simulink model "AVIC_model"  (R2015b)
settings: Solver=ode45  StartTime=0.0  StopTime=simtime  RelTol=1e-3
values from neighbouring files (symbols this model uses):
  A = 1    [simulation.m]
  a1 = 1    [simulation.m]
  a2 = 3    [simulation.m]
  a3 = 3    [simulation.m]
  Amp1 = Ampl/1000000    (= 134.217728)    [simulation.m]
  b1 = 1    [simulation.m]
  B2 = 8    [simulation.m]
  C = 32    [simulation.m]
  c1 = 1    [simulation.m]
  c2 = 1    [simulation.m]
  c3 = 1    [simulation.m]
  finrad = 2*pi/(N)*f0*clk    [simulation.m]
  FSC = 2^27    (= 134217728)    [simulation.m]
  SAT = 127    [simulation.m]
  Ts = 1/clk    (= 1.62760416667e-07)    [simulation.m]
libraries: simulink x298
(part 1 of 5)
settings Model: Creator=12x2123  LastModifiedBy=yuki
settings DataIOCC: SaveFormat=Array
settings HardwareCC: ProdBitPerPointer=32  ProdLargestAtomicFloat=None  ProdIntDivRoundTo=Undefined  ProdEndianess=Unspecified  ProdWordSize=32  ProdHWDeviceType=32-bit Generic
settings GRTTargetCC: GeneratePreprocessorConditionals=Disable all
settings ConfigComp: CovModelRefEnable=Off

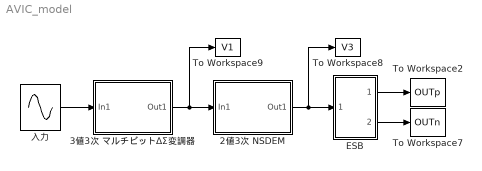
== system AVIC_model ==
  2値3次 NSDEM : Subsystem
  "3値3次 マルチビットΔΣ変調器 " : Subsystem
  ESB : Subsystem
  To Workspace2 : ToWorkspace  VariableName=OUTp  SampleTime=-1
  To Workspace7 : ToWorkspace  VariableName=OUTn  SampleTime=-1
  To Workspace8 : ToWorkspace  VariableName=V3  SampleTime=-1
  To Workspace9 : ToWorkspace  VariableName=V1  SampleTime=-1
  入力 : Sin  Amplitude=Amp1  Frequency=finrad  SampleTime=Ts
  wires:
  入力/1 -> "3値3次 マルチビットΔΣ変調器 "/1(In1)
  "3値3次 マルチビットΔΣ変調器 "/1(Out1) -> To Workspace9/1, 2値3次 NSDEM/1(In1)
  2値3次 NSDEM/1(Out1) -> ESB/1(In1), To Workspace8/1
  ESB/1(Out1) -> To Workspace2/1
  ESB/2(Out2) -> To Workspace7/1

== system AVIC_model/2値3次 NSDEM ==
  In1 : Inport
  NSDEM_3rd : Subsystem
  Out1 : Outport
  wires:
  NSDEM_3rd/1(OUT) -> Out1/1
  In1/1 -> NSDEM_3rd/1(IN)

== system AVIC_model/3値3次 マルチビットΔΣ変調器  ==
  In1 : Inport
  B1 : Gain  Gain=b1  SampleTime=Ts  SaturateOnIntegerOverflow=on  OutDataTypeStr=Inherit: Same as input  ParamDataTypeStr=Inherit: Same as input
  INT1 : Subsystem
  INT2 : Subsystem
  INT3 : Subsystem
  Q1 : Subsystem
  Scope3 : Scope  NumInputPorts=3
  To Workspace1 : ToWorkspace  VariableName=XN  SampleTime=-1
  To Workspace3 : ToWorkspace  VariableName=XN1  SampleTime=-1
  To Workspace4 : ToWorkspace  VariableName=XN2  SampleTime=-1
  To Workspace5 : ToWorkspace  VariableName=V  SampleTime=-1
  To Workspace6 : ToWorkspace  VariableName=Y  SampleTime=-1
  a1 : Gain  Gain=a1  OutDataTypeStr=Inherit: Same as input  ParamDataTypeStr=Inherit: Same as input
  a2 : Gain  Gain=a2  OutDataTypeStr=Inherit: Same as input  ParamDataTypeStr=Inherit: Same as input
  a3 : Gain  Gain=a3  OutDataTypeStr=Inherit: Same as input  ParamDataTypeStr=Inherit: Same as input
  c1 : Gain  Gain=c1  OutDataTypeStr=Inherit: Same as input  ParamDataTypeStr=Inherit: Same as input
  c2 : Gain  Gain=c2  OutDataTypeStr=Inherit: Same as input  ParamDataTypeStr=Inherit: Same as input
  c3 : Gain  Gain=c3  OutDataTypeStr=Inherit: Same as input  ParamDataTypeStr=Inherit: Same as input
  dd : Sum  Inputs=|+-  OutDataTypeStr=double  SaturateOnIntegerOverflow=on  InputSameDT=on
  dd1 : Sum  Inputs=|+-  OutDataTypeStr=double  SaturateOnIntegerOverflow=on  InputSameDT=on
  dd2 : Sum  Inputs=|+-  OutDataTypeStr=double  SaturateOnIntegerOverflow=on  InputSameDT=on
  Out1 : Outport
  wires:
  B1/1 -> dd1/1
  c1/1 -> dd/1
  INT1/1(Out1) -> c1/1, Scope3/1, To Workspace1/1
  a1/1 -> dd1/2
  dd/1 -> INT2/1(In1)
  a2/1 -> dd/2
  Q1/2(DA) -> Out1/1
  dd2/1 -> INT3/1(In1)
  INT2/1(Out1) -> To Workspace3/1, Scope3/2, c2/1
  Q1/1(Out1) -> a3/1, a2/1, a1/1, To Workspace5/1
  c3/1 -> To Workspace6/1, Q1/1(In1)
  dd1/1 -> INT1/1(In1)
  a3/1 -> dd2/2
  c2/1 -> dd2/1
  INT3/1(Out1) -> Scope3/3, To Workspace4/1, c3/1
  In1/1 -> B1/1

== system AVIC_model/ESB ==
  In1 : Inport
  Data Type Conversion2 : DataTypeConversion  OutDataTypeStr=double
  Data Type Conversion3 : DataTypeConversion  OutDataTypeStr=double
  Demux2 : Demux  Outputs=8
  Demux3 : Demux  Outputs=8
  Gain{17..32} (16 alike) : Gain
  Mux : Mux  Inputs=8
  Mux1 : Mux  Inputs=8
  Subsystem4 : Subsystem
  Out1 : Outport
  Out2 : Outport  Port=2
  wires:
  Subsystem4/1(Out1) -> Data Type Conversion2/1
  In1/1 -> Subsystem4/1(In1)
  Demux2/1 -> Gain18/1
  Demux2/2 -> Gain17/1
  Demux2/3 -> Gain20/1
  Demux2/4 -> Gain19/1
  Demux2/5 -> Gain22/1
  Demux2/6 -> Gain21/1
  Demux2/7 -> Gain24/1
  Demux2/8 -> Gain23/1
  Data Type Conversion2/1 -> Demux2/1
  Gain18/1 -> Mux/1
  Gain17/1 -> Mux/2
  Gain20/1 -> Mux/3
  Gain19/1 -> Mux/4
  Gain22/1 -> Mux/5
  Gain23/1 -> Mux/8
  Gain24/1 -> Mux/7
  Gain21/1 -> Mux/6
  Mux/1 -> Out1/1
  Subsystem4/2(Out2) -> Data Type Conversion3/1
  Demux3/1 -> Gain25/1
  Demux3/2 -> Gain32/1
  Demux3/3 -> Gain27/1
  Demux3/4 -> Gain26/1
  Demux3/5 -> Gain29/1
  Demux3/6 -> Gain28/1
  Demux3/7 -> Gain31/1
  Demux3/8 -> Gain30/1
  Data Type Conversion3/1 -> Demux3/1
  Gain25/1 -> Mux1/1
  Gain32/1 -> Mux1/2
  Gain27/1 -> Mux1/3
  Gain26/1 -> Mux1/4
  Gain29/1 -> Mux1/5
  Gain30/1 -> Mux1/8
  Gain31/1 -> Mux1/7
  Gain28/1 -> Mux1/6
  Mux1/1 -> Out2/1

== system AVIC_model/2値3次 NSDEM/NSDEM_3rd ==
  note: SORT8
  IN : Inport
  Data Type Conversion : DataTypeConversion  OutDataTypeStr=double
  Demux : Demux  Outputs=16
  INTEG4_1 : Subsystem
  INTEG4_10 : Subsystem
  INTEG4_11 : Subsystem
  INTEG4_12 : Subsystem
  INTEG4_13 : Subsystem
  INTEG4_14 : Subsystem
  INTEG4_15 : Subsystem
  INTEG4_17 : Subsystem
  INTEG4_2 : Subsystem
  INTEG4_3 : Subsystem
  INTEG4_4 : Subsystem
  INTEG4_5 : Subsystem
  INTEG4_6 : Subsystem
  INTEG4_7 : Subsystem
  INTEG4_8 : Subsystem
  INTEG4_9 : Subsystem
  MinMax : MinMax  Inputs=16
  MinMax1 : MinMax  Inputs=16
  SELECTOR1 : Subsystem
  Scope : Scope  NumInputPorts=16
  Scope1 : Scope  NumInputPorts=16
  Scope2 : Scope  NumInputPorts=16
  Sort16 : Subsystem
  To Workspace1 : ToWorkspace  VariableName=MIN3_1p  SampleTime=-1
  To Workspace2 : ToWorkspace  VariableName=IDX_1p  SampleTime=-1
  To Workspace5 : ToWorkspace  VariableName=MIN1_1p  SampleTime=-1
  To Workspace8 : ToWorkspace  VariableName=MIN2_1p  SampleTime=-1
  OUT : Outport
  wires:
  Sort16/2(IDX) -> To Workspace2/1, SELECTOR1/2(INX)
  Sort16/1(MIN) -> INTEG4_5/4(SUB3), INTEG4_6/4(SUB3), INTEG4_15/4(SUB3), INTEG4_14/4(SUB3), INTEG4_13/4(SUB3), INTEG4_12/4(SUB3), INTEG4_11/4(SUB3), INTEG4_10/4(SUB3), INTEG4_8/4(SUB3), INTEG4_9/4(SUB3), INTEG4_7/4(SUB3), INTEG4_4/4(SUB3), INTEG4_3/4(SUB3), INTEG4_1/4(SUB3), INTEG4_17/4(SUB3), INTEG4_2/4(SUB3), To Workspace1/1
  INTEG4_6/1(OUT1) -> Scope/7, MinMax/7
  INTEG4_5/1(OUT1) -> Scope/6, MinMax/6
  INTEG4_3/1(OUT1) -> Scope/4, MinMax/4
  INTEG4_2/1(OUT1) -> Scope/3, MinMax/3
  INTEG4_1/1(OUT1) -> Scope/2, MinMax/2
  INTEG4_17/1(OUT1) -> Scope/1, MinMax/1
  SELECTOR1/1(SEL) -> Data Type Conversion/1, OUT/1
  IN/1 -> SELECTOR1/1(TH)
  Demux/8 -> INTEG4_7/1(IN)
  Demux/7 -> INTEG4_6/1(IN)
  Demux/6 -> INTEG4_5/1(IN)
  Demux/5 -> INTEG4_4/1(IN)
  Demux/4 -> INTEG4_3/1(IN)
  Demux/3 -> INTEG4_2/1(IN)
  Demux/2 -> INTEG4_1/1(IN)
  Data Type Conversion/1 -> Demux/1
  MinMax1/1 -> INTEG4_17/3(SUB2), INTEG4_1/3(SUB2), INTEG4_2/3(SUB2), INTEG4_3/3(SUB2), INTEG4_4/3(SUB2), INTEG4_5/3(SUB2), INTEG4_6/3(SUB2), INTEG4_15/3(SUB2), INTEG4_14/3(SUB2), INTEG4_13/3(SUB2), INTEG4_12/3(SUB2), INTEG4_11/3(SUB2), INTEG4_10/3(SUB2), INTEG4_8/3(SUB2), INTEG4_9/3(SUB2), INTEG4_7/3(SUB2), To Workspace8/1
  INTEG4_4/1(OUT1) -> Scope/5, MinMax/5
  INTEG4_7/1(OUT1) -> Scope/8, MinMax/8
  Demux/1 -> INTEG4_17/1(IN)
  INTEG4_9/1(OUT1) -> Scope/9, MinMax/9
  INTEG4_8/1(OUT1) -> Scope/10, MinMax/10
  INTEG4_10/1(OUT1) -> Scope/11, MinMax/11
  INTEG4_11/1(OUT1) -> Scope/12, MinMax/12
  INTEG4_12/1(OUT1) -> Scope/13, MinMax/13
  INTEG4_13/1(OUT1) -> Scope/14, MinMax/14
  INTEG4_15/1(OUT1) -> Scope/16, MinMax/16
  Demux/9 -> INTEG4_9/1(IN)
  Demux/10 -> INTEG4_8/1(IN)
  Demux/11 -> INTEG4_10/1(IN)
  Demux/12 -> INTEG4_11/1(IN)
  Demux/16 -> INTEG4_15/1(IN)
  Demux/15 -> INTEG4_14/1(IN)
  Demux/14 -> INTEG4_13/1(IN)
  Demux/13 -> INTEG4_12/1(IN)
  MinMax/1 -> To Workspace5/1, INTEG4_17/2(SUB1), INTEG4_1/2(SUB1), INTEG4_2/2(SUB1), INTEG4_3/2(SUB1), INTEG4_4/2(SUB1), INTEG4_5/2(SUB1), INTEG4_6/2(SUB1), INTEG4_9/2(SUB1), INTEG4_8/2(SUB1), INTEG4_12/2(SUB1), INTEG4_14/2(SUB1), INTEG4_15/2(SUB1), INTEG4_13/2(SUB1), INTEG4_11/2(SUB1), INTEG4_10/2(SUB1), INTEG4_7/2(SUB1)
  INTEG4_14/1(OUT1) -> Scope/15, MinMax/15
  INTEG4_6/2(OUT2) -> Scope1/7, MinMax1/7
  INTEG4_5/2(OUT2) -> Scope1/6, MinMax1/6
  INTEG4_3/2(OUT2) -> Scope1/4, MinMax1/4
  INTEG4_2/2(OUT2) -> Scope1/3, MinMax1/3
  INTEG4_1/2(OUT2) -> Scope1/2, MinMax1/2
  INTEG4_17/2(OUT2) -> Scope1/1, MinMax1/1
  INTEG4_4/2(OUT2) -> Scope1/5, MinMax1/5
  INTEG4_7/2(OUT2) -> Scope1/8, MinMax1/8
  INTEG4_9/2(OUT2) -> Scope1/9, MinMax1/9
  INTEG4_8/2(OUT2) -> Scope1/10, MinMax1/10
  INTEG4_10/2(OUT2) -> Scope1/11, MinMax1/11
  INTEG4_11/2(OUT2) -> Scope1/12, MinMax1/12
  INTEG4_12/2(OUT2) -> Scope1/13, MinMax1/13
  INTEG4_13/2(OUT2) -> Scope1/14, MinMax1/14
  INTEG4_15/2(OUT2) -> Scope1/16, MinMax1/16
  INTEG4_14/2(OUT2) -> Scope1/15, MinMax1/15
  INTEG4_6/3(OUT3) -> Scope2/7, Sort16/7(IN6)
  INTEG4_5/3(OUT3) -> Scope2/6, Sort16/6(IN5)
  INTEG4_3/3(OUT3) -> Scope2/4, Sort16/4(IN3)
  INTEG4_2/3(OUT3) -> Scope2/3, Sort16/3(IN2)
  INTEG4_1/3(OUT3) -> Scope2/2, Sort16/2(IN1)
  INTEG4_17/3(OUT3) -> Scope2/1, Sort16/1(IN0)
  INTEG4_4/3(OUT3) -> Scope2/5, Sort16/5(IN4)
  INTEG4_7/3(OUT3) -> Scope2/8, Sort16/8(IN7)
  INTEG4_9/3(OUT3) -> Scope2/9, Sort16/9(IN8)
  INTEG4_8/3(OUT3) -> Scope2/10, Sort16/10(IN9)
  INTEG4_10/3(OUT3) -> Scope2/11, Sort16/11(IN10)
  INTEG4_11/3(OUT3) -> Scope2/12, Sort16/12(IN11)
  INTEG4_12/3(OUT3) -> Scope2/13, Sort16/13(IN12)
  INTEG4_13/3(OUT3) -> Scope2/14, Sort16/14(IN13)
  INTEG4_15/3(OUT3) -> Scope2/16, Sort16/16(IN15)
  INTEG4_14/3(OUT3) -> Scope2/15, Sort16/15(IN14)

== system AVIC_model/3値3次 マルチビットΔΣ変調器 /INT1 ==
  In1 : Inport
  INT1 : UnitDelay  SampleTime=Ts
  dd2 : Sum  Inputs=++|  OutDataTypeStr=double  SaturateOnIntegerOverflow=on  InputSameDT=on
  Out1 : Outport
  wires:
  dd2/1 -> INT1/1
  INT1/1 -> dd2/1, Out1/1
  In1/1 -> dd2/2

== system AVIC_model/3値3次 マルチビットΔΣ変調器 /INT2 ==
  In1 : Inport
  INT1 : UnitDelay  SampleTime=Ts
  dd2 : Sum  Inputs=++|  OutDataTypeStr=double  SaturateOnIntegerOverflow=on  InputSameDT=on
  Out1 : Outport
  wires:
  In1/1 -> dd2/2
  INT1/1 -> Out1/1, dd2/1
  dd2/1 -> INT1/1

== system AVIC_model/3値3次 マルチビットΔΣ変調器 /INT3 ==
  In1 : Inport
  INT1 : UnitDelay  SampleTime=Ts
  dd2 : Sum  Inputs=++|  OutDataTypeStr=double  SaturateOnIntegerOverflow=on  InputSameDT=on
  Out1 : Outport
  wires:
  dd2/1 -> INT1/1
  INT1/1 -> dd2/1, Out1/1
  In1/1 -> dd2/2

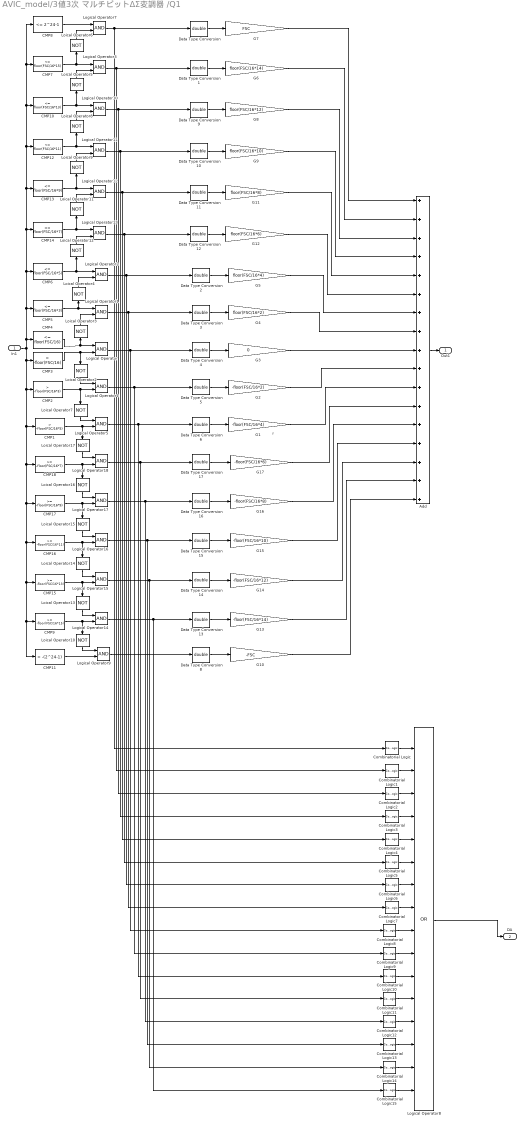
== system AVIC_model/3値3次 マルチビットΔΣ変調器 /Q1 ==
  note: f
  In1 : Inport
  Add : Sum  Inputs=+++++++++++++++++  OutDataTypeStr=double
  CMP1 : simulink/Logic and Bit Operations/Compare To Constant  relop=>  const=-floor(FSC/16*5)  OutDataTypeStr=boolean  ZeroCross=off
  CMP10 : simulink/Logic and Bit Operations/Compare To Constant  relop=<=  const=floor(FSC/16*13)  OutDataTypeStr=boolean  ZeroCross=off
  CMP11 : simulink/Logic and Bit Operations/Compare To Constant  relop=>  const=-(2^24-1)  OutDataTypeStr=boolean  ZeroCross=off
  CMP12 : simulink/Logic and Bit Operations/Compare To Constant  relop=<=  const=floor(FSC/16*11)  OutDataTypeStr=boolean  ZeroCross=off
  CMP13 : simulink/Logic and Bit Operations/Compare To Constant  relop=<=  const=floor(FSC/16*9)  OutDataTypeStr=boolean  ZeroCross=off
  CMP14 : simulink/Logic and Bit Operations/Compare To Constant  relop=<=  const=floor(FSC/16*7)  OutDataTypeStr=boolean  ZeroCross=off
  CMP15 : simulink/Logic and Bit Operations/Compare To Constant  relop=>=  const=-floor(FSC/16*13)  OutDataTypeStr=boolean  ZeroCross=off
  CMP16 : simulink/Logic and Bit Operations/Compare To Constant  relop=>=  const=-floor(FSC/16*11)  OutDataTypeStr=boolean  ZeroCross=off
  CMP17 : simulink/Logic and Bit Operations/Compare To Constant  relop=>=  const=-floor(FSC/16*9)  OutDataTypeStr=boolean  ZeroCross=off
  CMP18 : simulink/Logic and Bit Operations/Compare To Constant  relop=>=  const=-floor(FSC/16*7)  OutDataTypeStr=boolean  ZeroCross=off
  CMP2 : simulink/Logic and Bit Operations/Compare To Constant  relop=>  const=-floor(FSC/16*3)  OutDataTypeStr=boolean  ZeroCross=off
  CMP3 : simulink/Logic and Bit Operations/Compare To Constant  relop=>  const=-floor(FSC/16)  OutDataTypeStr=boolean  ZeroCross=off
  CMP4 : simulink/Logic and Bit Operations/Compare To Constant  relop=<=  const=floor(FSC/16)  OutDataTypeStr=boolean  ZeroCross=off
  CMP5 : simulink/Logic and Bit Operations/Compare To Constant  relop=<=  const=floor(FSC/16*3)  OutDataTypeStr=boolean  ZeroCross=off
  CMP6 : simulink/Logic and Bit Operations/Compare To Constant  relop=<=  const=floor(FSC/16*5)  OutDataTypeStr=boolean  ZeroCross=off
  CMP7 : simulink/Logic and Bit Operations/Compare To Constant  relop=<=  const=floor(FSC/16*15)  OutDataTypeStr=boolean  ZeroCross=off
  CMP8 : simulink/Logic and Bit Operations/Compare To Constant  relop=<=  const=2^24-1  OutDataTypeStr=boolean  ZeroCross=off
  CMP9 : simulink/Logic and Bit Operations/Compare To Constant  relop=>=  const=-floor(FSC/16*15)  OutDataTypeStr=boolean  ZeroCross=off
  Combinatorial Logic : CombinatorialLogic  TruthTable=[0 0 0 0 0 0 0 0 0 0 0 0 0 0 0 0;1 1 1 1 1 1 1 1 1 1 1 1 1 1 1 1]
  Combinatorial Logic1 : CombinatorialLogic  TruthTable=[0 0 0 0 0 0 0 0 0 0 0 0 0 0 0 0;1 1 1 1 1 1 1 1 1 1 1 1 1 1 1 0]
  Combinatorial Logic10 : CombinatorialLogic  TruthTable=[0 0 0 0 0 0 0 0 0 0 0 0 0 0 0 0;1 1 1 1 1 1 0 0 0 0 0 0 0 0 0 0]
  Combinatorial Logic11 : CombinatorialLogic  TruthTable=[0 0 0 0 0 0 0 0 0 0 0 0 0 0 0 0;1 1 1 1 1 0 0 0 0 0 0 0 0 0 0 0]
  Combinatorial Logic12 : CombinatorialLogic  TruthTable=[0 0 0 0 0 0 0 0 0 0 0 0 0 0 0 0;1 1 1 1 0 0 0 0 0 0 0 0 0 0 0 0]
  Combinatorial Logic13 : CombinatorialLogic  TruthTable=[0 0 0 0 0 0 0 0 0 0 0 0 0 0 0 0;1 1 1 0 0 0 0 0 0 0 0 0 0 0 0 0]
  Combinatorial Logic14 : CombinatorialLogic  TruthTable=[0 0 0 0 0 0 0 0 0 0 0 0 0 0 0 0;1 1 0 0 0 0 0 0 0 0 0 0 0 0 0 0]
  Combinatorial Logic15 : CombinatorialLogic  TruthTable=[0 0 0 0 0 0 0 0 0 0 0 0 0 0 0 0;1 0 0 0 0 0 0 0 0 0 0 0 0 0 0 0]
  Combinatorial Logic2 : CombinatorialLogic  TruthTable=[0 0 0 0 0 0 0 0 0 0 0 0 0 0 0 0;1 1 1 1 1 1 1 1 1 1 1 1 1 1 0 0]
  Combinatorial Logic3 : CombinatorialLogic  TruthTable=[0 0 0 0 0 0 0 0 0 0 0 0 0 0 0 0;1 1 1 1 1 1 1 1 1 1 1 1 1 0 0 0]
  Combinatorial Logic4 : CombinatorialLogic  TruthTable=[0 0 0 0 0 0 0 0 0 0 0 0 0 0 0 0;1 1 1 1 1 1 1 1 1 1 1 1 0 0 0 0]
  Combinatorial Logic5 : CombinatorialLogic  TruthTable=[0 0 0 0 0 0 0 0 0 0 0 0 0 0 0 0;1 1 1 1 1 1 1 1 1 1 1 0 0 0 0 0]
  Combinatorial Logic6 : CombinatorialLogic  TruthTable=[0 0 0 0 0 0 0 0 0 0 0 0 0 0 0 0;1 1 1 1 1 1 1 1 1 1 0 0 0 0 0 0]
  Combinatorial Logic7 : CombinatorialLogic  TruthTable=[0 0 0 0 0 0 0 0 0 0 0 0 0 0 0 0;1 1 1 1 1 1 1 1 1 0 0 0 0 0 0 0]
  Combinatorial Logic8 : CombinatorialLogic  TruthTable=[0 0 0 0 0 0 0 0 0 0 0 0 0 0 0 0;1 1 1 1 1 1 1 1 0 0 0 0 0 0 0 0]
  Combinatorial Logic9 : CombinatorialLogic  TruthTable=[0 0 0 0 0 0 0 0 0 0 0 0 0 0 0 0;1 1 1 1 1 1 1 0 0 0 0 0 0 0 0 0]
  Data Type Conversion{,1..6,8..17} (17 alike) : DataTypeConversion  OutDataTypeStr=double
  G1 : Gain  Gain=-floor(FSC/16*4)  OutDataTypeStr=Inherit: Same as input  ParamDataTypeStr=Inherit: Same as input
  G10 : Gain  Gain=-FSC  OutDataTypeStr=Inherit: Same as input  ParamDataTypeStr=Inherit: Same as input
  G11 : Gain  Gain=floor(FSC/16*8)  OutDataTypeStr=Inherit: Same as input  ParamDataTypeStr=Inherit: Same as input
  G12 : Gain  Gain=floor(FSC/16*6)  OutDataTypeStr=Inherit: Same as input  ParamDataTypeStr=Inherit: Same as input
  G13 : Gain  Gain=-floor(FSC/16*14)  OutDataTypeStr=Inherit: Same as input  ParamDataTypeStr=Inherit: Same as input
  G14 : Gain  Gain=-floor(FSC/16*12)  OutDataTypeStr=Inherit: Same as input  ParamDataTypeStr=Inherit: Same as input
  G15 : Gain  Gain=-floor(FSC/16*10)  OutDataTypeStr=Inherit: Same as input  ParamDataTypeStr=Inherit: Same as input
  G16 : Gain  Gain=-floor(FSC/16*8)  OutDataTypeStr=Inherit: Same as input  ParamDataTypeStr=Inherit: Same as input
  G17 : Gain  Gain=-floor(FSC/16*6)  OutDataTypeStr=Inherit: Same as input  ParamDataTypeStr=Inherit: Same as input
  G2 : Gain  Gain=-floor(FSC/16*2)  OutDataTypeStr=Inherit: Same as input  ParamDataTypeStr=Inherit: Same as input
  G3 : Gain  Gain=0  OutDataTypeStr=Inherit: Same as input  ParamDataTypeStr=Inherit: Same as input
  G4 : Gain  Gain=floor(FSC/16*2)  OutDataTypeStr=Inherit: Same as input  ParamDataTypeStr=Inherit: Same as input
  G5 : Gain  Gain=floor(FSC/16*4)  OutDataTypeStr=Inherit: Same as input  ParamDataTypeStr=Inherit: Same as input
  G6 : Gain  Gain=floor(FSC/16*14)  OutDataTypeStr=Inherit: Same as input  ParamDataTypeStr=Inherit: Same as input
  G7 : Gain  Gain=FSC  OutDataTypeStr=Inherit: Same as input  ParamDataTypeStr=Inherit: Same as input
  G8 : Gain  Gain=floor(FSC/16*12)  OutDataTypeStr=Inherit: Same as input  ParamDataTypeStr=Inherit: Same as input
  G9 : Gain  Gain=floor(FSC/16*10)  OutDataTypeStr=Inherit: Same as input  ParamDataTypeStr=Inherit: Same as input
  Logical Operator{,1..5,7,9..18} (17 alike) : Logic  AllPortsSameDT=off  OutDataTypeStr=boolean
  Logical Operator8 : Logic  Operator=OR  Inputs=16  AllPortsSameDT=off  OutDataTypeStr=boolean
  Loical Operator{2..17} (16 alike) : Logic  Operator=NOT  AllPortsSameDT=off  OutDataTypeStr=boolean
  Out1 : Outport
  DA : Outport  Port=2
  wires:
  Combinatorial Logic8/1 -> Logical Operator8/9
  Combinatorial Logic9/1 -> Logical Operator8/10
  Combinatorial Logic10/1 -> Logical Operator8/11
  Combinatorial Logic11/1 -> Logical Operator8/12
  Combinatorial Logic12/1 -> Logical Operator8/13
  Combinatorial Logic13/1 -> Logical Operator8/14
  Combinatorial Logic14/1 -> Logical Operator8/15
  Combinatorial Logic15/1 -> Logical Operator8/16
  Logical Operator8/1 -> DA/1
  Combinatorial Logic/1 -> Logical Operator8/1
  Combinatorial Logic1/1 -> Logical Operator8/2
  Combinatorial Logic2/1 -> Logical Operator8/3
  Combinatorial Logic3/1 -> Logical Operator8/4
  Combinatorial Logic4/1 -> Logical Operator8/5
  Combinatorial Logic5/1 -> Logical Operator8/6
  Combinatorial Logic6/1 -> Logical Operator8/7
  Combinatorial Logic7/1 -> Logical Operator8/8
  G10/1 -> Add/17
  G13/1 -> Add/16
  G14/1 -> Add/15
  G15/1 -> Add/14
  G16/1 -> Add/13
  G17/1 -> Add/12
  G1/1 -> Add/11
  G2/1 -> Add/10
  G3/1 -> Add/9
  G4/1 -> Add/8
  G5/1 -> Add/7
  G12/1 -> Add/6
  G11/1 -> Add/5
  G9/1 -> Add/4
  G8/1 -> Add/3
  G6/1 -> Add/2
  G7/1 -> Add/1
  Data Type Conversion17/1 -> G17/1
  CMP18/1 -> Loical Operator16/1, Logical Operator18/2
  Logical Operator18/1 -> Combinatorial Logic11/1, Data Type Conversion17/1
  Loical Operator17/1 -> Logical Operator18/1
  Data Type Conversion16/1 -> G16/1
  CMP17/1 -> Loical Operator15/1, Logical Operator17/2
  Logical Operator17/1 -> Combinatorial Logic12/1, Data Type Conversion16/1
  Loical Operator16/1 -> Logical Operator17/1
  Data Type Conversion15/1 -> G15/1
  CMP16/1 -> Loical Operator14/1, Logical Operator16/2
  Logical Operator16/1 -> Data Type Conversion15/1, Combinatorial Logic13/1
  Loical Operator15/1 -> Logical Operator16/1
  Data Type Conversion14/1 -> G14/1
  CMP15/1 -> Loical Operator13/1, Logical Operator15/2
  Logical Operator15/1 -> Combinatorial Logic14/1, Data Type Conversion14/1
  Loical Operator14/1 -> Logical Operator15/1
  Data Type Conversion13/1 -> G13/1
  CMP9/1 -> Loical Operator10/1, Logical Operator14/2
  Logical Operator14/1 -> Combinatorial Logic15/1, Data Type Conversion13/1
  Loical Operator13/1 -> Logical Operator14/1
  Data Type Conversion8/1 -> G10/1
  CMP11/1 -> Logical Operator9/2
  Logical Operator9/1 -> Data Type Conversion8/1
  Loical Operator10/1 -> Logical Operator9/1
  Data Type Conversion12/1 -> G12/1
  Logical Operator13/1 -> Combinatorial Logic5/1, Data Type Conversion12/1
  Loical Operator12/1 -> Logical Operator13/2
  CMP14/1 -> Loical Operator11/1, Logical Operator13/1
  Data Type Conversion11/1 -> G11/1
  Logical Operator12/1 -> Combinatorial Logic4/1, Data Type Conversion11/1
  Loical Operator11/1 -> Logical Operator12/2
  CMP13/1 -> Loical Operator9/1, Logical Operator12/1
  Data Type Conversion10/1 -> G9/1
  Logical Operator11/1 -> Combinatorial Logic3/1, Data Type Conversion10/1
  Loical Operator9/1 -> Logical Operator11/2
  CMP12/1 -> Loical Operator8/1, Logical Operator11/1
  Data Type Conversion9/1 -> G8/1
  Logical Operator10/1 -> Combinatorial Logic2/1, Data Type Conversion9/1
  Loical Operator8/1 -> Logical Operator10/2
  CMP10/1 -> Loical Operator5/1, Logical Operator10/1
  Add/1 -> Out1/1
  Data Type Conversion6/1 -> G1/1
  Data Type Conversion5/1 -> G2/1
  Data Type Conversion4/1 -> G3/1
  Data Type Conversion3/1 -> G4/1
  Data Type Conversion2/1 -> G5/1
  Data Type Conversion1/1 -> G6/1
  Data Type Conversion/1 -> G7/1
  Logical Operator7/1 -> Combinatorial Logic/1, Data Type Conversion/1
  Loical Operator6/1 -> Logical Operator7/2
  CMP8/1 -> Logical Operator7/1
  In1/1 -> CMP9/1, CMP11/1, CMP15/1, CMP16/1, CMP17/1, CMP18/1, CMP1/1, CMP2/1, CMP3/1, CMP4/1, CMP7/1, CMP8/1, CMP10/1, CMP12/1, CMP13/1, CMP14/1, CMP6/1, CMP5/1
  CMP3/1 -> Logical Operator/2, Loical Operator2/1
  CMP2/1 -> Logical Operator4/2, Loical Operator7/1
  CMP1/1 -> Loical Operator17/1, Logical Operator5/2
  Logical Operator3/1 -> Combinatorial Logic1/1, Data Type Conversion1/1
  Logical Operator2/1 -> Combinatorial Logic6/1, Data Type Conversion2/1
  Logical Operator1/1 -> Combinatorial Logic7/1, Data Type Conversion3/1
  Logical Operator/1 -> Combinatorial Logic8/1, Data Type Conversion4/1
  Logical Operator4/1 -> Combinatorial Logic9/1, Data Type Conversion5/1
  Logical Operator5/1 -> Combinatorial Logic10/1, Data Type Conversion6/1
  Loical Operator7/1 -> Logical Operator5/1
  Loical Operator2/1 -> Logical Operator4/1
  CMP4/1 -> Logical Operator/1, Loical Operator3/1
  Loical Operator3/1 -> Logical Operator1/2
  CMP5/1 -> Logical Operator1/1, Loical Operator4/1
  Loical Operator4/1 -> Logical Operator2/2
  CMP6/1 -> Loical Operator12/1, Logical Operator2/1
  Loical Operator5/1 -> Logical Operator3/2
  CMP7/1 -> Loical Operator6/1, Logical Operator3/1

== system AVIC_model/ESB/Subsystem4 ==
  In1 : Inport
  Demux : Demux  Outputs=16
  Logical Operator : Logic  Operator=OR  Inputs=8  AllPortsSameDT=off  OutDataTypeStr=boolean
  Logical Operator1 : Logic  Operator=OR  Inputs=8  AllPortsSameDT=off  OutDataTypeStr=boolean
  Subsystem : Subsystem
  Subsystem1 : Subsystem
  Subsystem2 : Subsystem
  Subsystem3 : Subsystem
  Subsystem4 : Subsystem
  Subsystem5 : Subsystem
  Subsystem6 : Subsystem
  Subsystem7 : Subsystem
  Sum{,1..7} (8 alike) : Sum
  To Workspace2 : ToWorkspace  VariableName=OUTp1  SampleTime=-1
  To Workspace7 : ToWorkspace  VariableName=OUTn1  SampleTime=-1
  Out1 : Outport
  Out2 : Outport  Port=2
  wires:
  In1/1 -> Demux/1
  Logical Operator/1 -> Out1/1
  Logical Operator1/1 -> Out2/1
  Sum1/1 -> Subsystem1/1(In1)
  Sum2/1 -> Subsystem2/1(In1)
  Sum/1 -> Subsystem/1(In1)
  Sum3/1 -> Subsystem3/1(In1)
  Sum5/1 -> Subsystem5/1(In1)
  Sum6/1 -> Subsystem6/1(In1)
  Sum4/1 -> Subsystem4/1(In1)
  Sum7/1 -> Subsystem7/1(In1)
  Demux/1 -> Sum/1
  Demux/2 -> Sum/2
  Demux/3 -> Sum1/1
  Demux/4 -> Sum1/2
  Demux/5 -> Sum2/1
  Demux/6 -> Sum2/2
  Demux/7 -> Sum3/1
  Demux/8 -> Sum3/2
  Demux/9 -> Sum4/1
  Demux/10 -> Sum4/2
  Demux/11 -> Sum5/1
  Demux/12 -> Sum5/2
  Demux/13 -> Sum6/1
  Demux/14 -> Sum6/2
  Demux/15 -> Sum7/1
  Demux/16 -> Sum7/2
  Subsystem/1("P1 ") -> Logical Operator/1, To Workspace2/1
  Subsystem1/1("P1 ") -> Logical Operator/2
  Subsystem2/1("P1 ") -> Logical Operator/3
  Subsystem3/1("P1 ") -> Logical Operator/4
  Subsystem4/1("P1 ") -> Logical Operator/5
  Subsystem5/1("P1 ") -> Logical Operator/6
  Subsystem6/1("P1 ") -> Logical Operator/7
  Subsystem7/1("P1 ") -> Logical Operator/8
  Subsystem/2("N1 ") -> To Workspace7/1, Logical Operator1/1
  Subsystem1/2("N1 ") -> Logical Operator1/2
  Subsystem2/2("N1 ") -> Logical Operator1/3
  Subsystem3/2("N1 ") -> Logical Operator1/4
  Subsystem4/2("N1 ") -> Logical Operator1/5
  Subsystem5/2("N1 ") -> Logical Operator1/6
  Subsystem6/2("N1 ") -> Logical Operator1/7
  Subsystem7/2("N1 ") -> Logical Operator1/8

== system AVIC_model/2値3次 NSDEM/NSDEM_3rd/INTEG4_1 ==
  IN : Inport
  SUB1 : Inport  Port=2
  SUB2 : Inport  Port=3
  SUB3 : Inport  Port=4
  Add{1..5} (5 alike) : Sum  Inputs=++-
  Gain : Gain  Gain=B2
  Gain1 : Gain  Gain=A
  Gain2 : Gain  Gain=C
  INT1 : UnitDelay  SampleTime=Ts
  INT2 : UnitDelay  SampleTime=Ts
  INT3 : UnitDelay  SampleTime=Ts
  Saturation{,1..4} (5 alike) : Saturate  UpperLimit=SAT  LowerLimit=-SAT
  OUT1 : Outport
  OUT2 : Outport  Port=2
  OUT3 : Outport  Port=3
  wires:
  SUB3/1 -> Add2/3
  INT1/1 -> Add2/1, OUT3/1
  INT2/1 -> OUT1/1, Add4/1, Add1/2
  Add4/1 -> Saturation/1
  SUB1/1 -> Add4/3, Add1/3
  IN/1 -> Gain/1, Gain2/1, Gain1/1
  Add1/1 -> Saturation1/1
  Gain/1 -> Add1/1
  Add2/1 -> Saturation2/1
  Saturation/1 -> INT2/1
  Saturation2/1 -> INT1/1
  INT3/1 -> OUT2/1, Add5/1, Add3/2
  Add5/1 -> Saturation3/1
  SUB2/1 -> Add5/3, Add3/3
  Add3/1 -> Saturation4/1
  Gain2/1 -> Add3/1
  Saturation3/1 -> INT3/1
  Saturation4/1 -> Add2/2
  Saturation1/1 -> Add5/2
  Gain1/1 -> Add4/2

== system AVIC_model/2値3次 NSDEM/NSDEM_3rd/INTEG4_10 ==
  IN : Inport
  SUB1 : Inport  Port=2
  SUB2 : Inport  Port=3
  SUB3 : Inport  Port=4
  Add{1..5} (5 alike) : Sum  Inputs=++-
  Gain : Gain  Gain=B2
  Gain1 : Gain  Gain=A
  Gain2 : Gain  Gain=C
  INT1 : UnitDelay  SampleTime=Ts
  INT2 : UnitDelay  SampleTime=Ts
  INT3 : UnitDelay  SampleTime=Ts
  Saturation{,1..4} (5 alike) : Saturate  UpperLimit=SAT  LowerLimit=-SAT
  OUT1 : Outport
  OUT2 : Outport  Port=2
  OUT3 : Outport  Port=3
  wires:
  SUB3/1 -> Add2/3
  INT1/1 -> Add2/1, OUT3/1
  INT2/1 -> OUT1/1, Add4/1, Add1/2
  Add4/1 -> Saturation/1
  SUB1/1 -> Add4/3, Add1/3
  IN/1 -> Gain/1, Gain2/1, Gain1/1
  Add1/1 -> Saturation1/1
  Gain/1 -> Add1/1
  Add2/1 -> Saturation2/1
  Saturation/1 -> INT2/1
  Saturation2/1 -> INT1/1
  INT3/1 -> OUT2/1, Add5/1, Add3/2
  Add5/1 -> Saturation3/1
  SUB2/1 -> Add5/3, Add3/3
  Add3/1 -> Saturation4/1
  Gain2/1 -> Add3/1
  Saturation3/1 -> INT3/1
  Saturation4/1 -> Add2/2
  Saturation1/1 -> Add5/2
  Gain1/1 -> Add4/2

== system AVIC_model/2値3次 NSDEM/NSDEM_3rd/INTEG4_11 ==
  IN : Inport
  SUB1 : Inport  Port=2
  SUB2 : Inport  Port=3
  SUB3 : Inport  Port=4
  Add{1..5} (5 alike) : Sum  Inputs=++-
  Gain : Gain  Gain=B2
  Gain1 : Gain  Gain=A
  Gain2 : Gain  Gain=C
  INT1 : UnitDelay  SampleTime=Ts
  INT2 : UnitDelay  SampleTime=Ts
  INT3 : UnitDelay  SampleTime=Ts
  Saturation{,1..4} (5 alike) : Saturate  UpperLimit=SAT  LowerLimit=-SAT
  OUT1 : Outport
  OUT2 : Outport  Port=2
  OUT3 : Outport  Port=3
  wires:
  SUB3/1 -> Add2/3
  INT1/1 -> Add2/1, OUT3/1
  INT2/1 -> OUT1/1, Add4/1, Add1/2
  Add4/1 -> Saturation/1
  SUB1/1 -> Add4/3, Add1/3
  IN/1 -> Gain/1, Gain2/1, Gain1/1
  Add1/1 -> Saturation1/1
  Gain/1 -> Add1/1
  Add2/1 -> Saturation2/1
  Saturation/1 -> INT2/1
  Saturation2/1 -> INT1/1
  INT3/1 -> OUT2/1, Add5/1, Add3/2
  Add5/1 -> Saturation3/1
  SUB2/1 -> Add5/3, Add3/3
  Add3/1 -> Saturation4/1
  Gain2/1 -> Add3/1
  Saturation3/1 -> INT3/1
  Saturation4/1 -> Add2/2
  Saturation1/1 -> Add5/2
  Gain1/1 -> Add4/2

== system AVIC_model/2値3次 NSDEM/NSDEM_3rd/INTEG4_12 ==
  IN : Inport
  SUB1 : Inport  Port=2
  SUB2 : Inport  Port=3
  SUB3 : Inport  Port=4
  Add{1..5} (5 alike) : Sum  Inputs=++-
  Gain : Gain  Gain=B2
  Gain1 : Gain  Gain=A
  Gain2 : Gain  Gain=C
  INT1 : UnitDelay  SampleTime=Ts
  INT2 : UnitDelay  SampleTime=Ts
  INT3 : UnitDelay  SampleTime=Ts
  Saturation{,1..4} (5 alike) : Saturate  UpperLimit=SAT  LowerLimit=-SAT
  OUT1 : Outport
  OUT2 : Outport  Port=2
  OUT3 : Outport  Port=3
  wires:
  SUB3/1 -> Add2/3
  INT1/1 -> Add2/1, OUT3/1
  INT2/1 -> OUT1/1, Add4/1, Add1/2
  Add4/1 -> Saturation/1
  SUB1/1 -> Add4/3, Add1/3
  IN/1 -> Gain/1, Gain2/1, Gain1/1
  Add1/1 -> Saturation1/1
  Gain/1 -> Add1/1
  Add2/1 -> Saturation2/1
  Saturation/1 -> INT2/1
  Saturation2/1 -> INT1/1
  INT3/1 -> OUT2/1, Add5/1, Add3/2
  Add5/1 -> Saturation3/1
  SUB2/1 -> Add5/3, Add3/3
  Add3/1 -> Saturation4/1
  Gain2/1 -> Add3/1
  Saturation3/1 -> INT3/1
  Saturation4/1 -> Add2/2
  Saturation1/1 -> Add5/2
  Gain1/1 -> Add4/2

== system AVIC_model/2値3次 NSDEM/NSDEM_3rd/INTEG4_13 ==
  IN : Inport
  SUB1 : Inport  Port=2
  SUB2 : Inport  Port=3
  SUB3 : Inport  Port=4
  Add{1..5} (5 alike) : Sum  Inputs=++-
  Gain : Gain  Gain=B2
  Gain1 : Gain  Gain=A
  Gain2 : Gain  Gain=C
  INT1 : UnitDelay  SampleTime=Ts
  INT2 : UnitDelay  SampleTime=Ts
  INT3 : UnitDelay  SampleTime=Ts
  Saturation{,1..4} (5 alike) : Saturate  UpperLimit=SAT  LowerLimit=-SAT
  OUT1 : Outport
  OUT2 : Outport  Port=2
  OUT3 : Outport  Port=3
  wires:
  SUB3/1 -> Add2/3
  INT1/1 -> Add2/1, OUT3/1
  INT2/1 -> OUT1/1, Add4/1, Add1/2
  Add4/1 -> Saturation/1
  SUB1/1 -> Add4/3, Add1/3
  IN/1 -> Gain/1, Gain2/1, Gain1/1
  Add1/1 -> Saturation1/1
  Gain/1 -> Add1/1
  Add2/1 -> Saturation2/1
  Saturation/1 -> INT2/1
  Saturation2/1 -> INT1/1
  INT3/1 -> OUT2/1, Add5/1, Add3/2
  Add5/1 -> Saturation3/1
  SUB2/1 -> Add5/3, Add3/3
  Add3/1 -> Saturation4/1
  Gain2/1 -> Add3/1
  Saturation3/1 -> INT3/1
  Saturation4/1 -> Add2/2
  Saturation1/1 -> Add5/2
  Gain1/1 -> Add4/2

== system AVIC_model/2値3次 NSDEM/NSDEM_3rd/INTEG4_14 ==
  IN : Inport
  SUB1 : Inport  Port=2
  SUB2 : Inport  Port=3
  SUB3 : Inport  Port=4
  Add{1..5} (5 alike) : Sum  Inputs=++-
  Gain : Gain  Gain=B2
  Gain1 : Gain  Gain=A
  Gain2 : Gain  Gain=C
  INT1 : UnitDelay  SampleTime=Ts
  INT2 : UnitDelay  SampleTime=Ts
  INT3 : UnitDelay  SampleTime=Ts
  Saturation{,1..4} (5 alike) : Saturate  UpperLimit=SAT  LowerLimit=-SAT
  OUT1 : Outport
  OUT2 : Outport  Port=2
  OUT3 : Outport  Port=3
  wires:
  SUB3/1 -> Add2/3
  INT1/1 -> Add2/1, OUT3/1
  INT2/1 -> OUT1/1, Add4/1, Add1/2
  Add4/1 -> Saturation/1
  SUB1/1 -> Add4/3, Add1/3
  IN/1 -> Gain/1, Gain2/1, Gain1/1
  Add1/1 -> Saturation1/1
  Gain/1 -> Add1/1
  Add2/1 -> Saturation2/1
  Saturation/1 -> INT2/1
  Saturation2/1 -> INT1/1
  INT3/1 -> OUT2/1, Add5/1, Add3/2
  Add5/1 -> Saturation3/1
  SUB2/1 -> Add5/3, Add3/3
  Add3/1 -> Saturation4/1
  Gain2/1 -> Add3/1
  Saturation3/1 -> INT3/1
  Saturation4/1 -> Add2/2
  Saturation1/1 -> Add5/2
  Gain1/1 -> Add4/2

== system AVIC_model/2値3次 NSDEM/NSDEM_3rd/INTEG4_15 ==
  IN : Inport
  SUB1 : Inport  Port=2
  SUB2 : Inport  Port=3
  SUB3 : Inport  Port=4
  Add{1..5} (5 alike) : Sum  Inputs=++-
  Gain : Gain  Gain=B2
  Gain1 : Gain  Gain=A
  Gain2 : Gain  Gain=C
  INT1 : UnitDelay  SampleTime=Ts
  INT2 : UnitDelay  SampleTime=Ts
  INT3 : UnitDelay  SampleTime=Ts
  Saturation{,1..4} (5 alike) : Saturate  UpperLimit=SAT  LowerLimit=-SAT
  OUT1 : Outport
  OUT2 : Outport  Port=2
  OUT3 : Outport  Port=3
  wires:
  SUB3/1 -> Add2/3
  INT1/1 -> Add2/1, OUT3/1
  INT2/1 -> OUT1/1, Add4/1, Add1/2
  Add4/1 -> Saturation/1
  SUB1/1 -> Add4/3, Add1/3
  IN/1 -> Gain/1, Gain2/1, Gain1/1
  Add1/1 -> Saturation1/1
  Gain/1 -> Add1/1
  Add2/1 -> Saturation2/1
  Saturation/1 -> INT2/1
  Saturation2/1 -> INT1/1
  INT3/1 -> OUT2/1, Add5/1, Add3/2
  Add5/1 -> Saturation3/1
  SUB2/1 -> Add5/3, Add3/3
  Add3/1 -> Saturation4/1
  Gain2/1 -> Add3/1
  Saturation3/1 -> INT3/1
  Saturation4/1 -> Add2/2
  Saturation1/1 -> Add5/2
  Gain1/1 -> Add4/2

== system AVIC_model/2値3次 NSDEM/NSDEM_3rd/INTEG4_17 ==
  IN : Inport
  SUB1 : Inport  Port=2
  SUB2 : Inport  Port=3
  SUB3 : Inport  Port=4
  Add{1..5} (5 alike) : Sum  Inputs=++-
  Gain : Gain  Gain=B2
  Gain1 : Gain  Gain=A
  Gain2 : Gain  Gain=C
  INT1 : UnitDelay  SampleTime=Ts
  INT2 : UnitDelay  SampleTime=Ts
  INT3 : UnitDelay  SampleTime=Ts
  Saturation{,1..4} (5 alike) : Saturate  UpperLimit=SAT  LowerLimit=-SAT
  OUT1 : Outport
  OUT2 : Outport  Port=2
  OUT3 : Outport  Port=3
  wires:
  SUB3/1 -> Add2/3
  INT1/1 -> Add2/1, OUT3/1
  INT2/1 -> OUT1/1, Add4/1, Add1/2
  Add4/1 -> Saturation/1
  SUB1/1 -> Add4/3, Add1/3
  IN/1 -> Gain/1, Gain2/1, Gain1/1
  Add1/1 -> Saturation1/1
  Gain/1 -> Add1/1
  Add2/1 -> Saturation2/1
  Saturation/1 -> INT2/1
  Saturation2/1 -> INT1/1
  INT3/1 -> OUT2/1, Add5/1, Add3/2
  Add5/1 -> Saturation3/1
  SUB2/1 -> Add5/3, Add3/3
  Add3/1 -> Saturation4/1
  Gain2/1 -> Add3/1
  Saturation3/1 -> INT3/1
  Saturation4/1 -> Add2/2
  Saturation1/1 -> Add5/2
  Gain1/1 -> Add4/2

== system AVIC_model/2値3次 NSDEM/NSDEM_3rd/INTEG4_2 ==
  IN : Inport
  SUB1 : Inport  Port=2
  SUB2 : Inport  Port=3
  SUB3 : Inport  Port=4
  Add{1..5} (5 alike) : Sum  Inputs=++-
  Gain : Gain  Gain=B2
  Gain1 : Gain  Gain=A
  Gain2 : Gain  Gain=C
  INT1 : UnitDelay  SampleTime=Ts
  INT2 : UnitDelay  SampleTime=Ts
  INT3 : UnitDelay  SampleTime=Ts
  Saturation{,1..4} (5 alike) : Saturate  UpperLimit=SAT  LowerLimit=-SAT
  OUT1 : Outport
  OUT2 : Outport  Port=2
  OUT3 : Outport  Port=3
  wires:
  SUB3/1 -> Add2/3
  INT1/1 -> Add2/1, OUT3/1
  INT2/1 -> OUT1/1, Add4/1, Add1/2
  Add4/1 -> Saturation/1
  SUB1/1 -> Add4/3, Add1/3
  IN/1 -> Gain/1, Gain2/1, Gain1/1
  Add1/1 -> Saturation1/1
  Gain/1 -> Add1/1
  Add2/1 -> Saturation2/1
  Saturation/1 -> INT2/1
  Saturation2/1 -> INT1/1
  INT3/1 -> OUT2/1, Add5/1, Add3/2
  Add5/1 -> Saturation3/1
  SUB2/1 -> Add5/3, Add3/3
  Add3/1 -> Saturation4/1
  Gain2/1 -> Add3/1
  Saturation3/1 -> INT3/1
  Saturation4/1 -> Add2/2
  Saturation1/1 -> Add5/2
  Gain1/1 -> Add4/2

== system AVIC_model/2値3次 NSDEM/NSDEM_3rd/INTEG4_3 ==
  IN : Inport
  SUB1 : Inport  Port=2
  SUB2 : Inport  Port=3
  SUB3 : Inport  Port=4
  Add{1..5} (5 alike) : Sum  Inputs=++-
  Gain : Gain  Gain=B2
  Gain1 : Gain  Gain=A
  Gain2 : Gain  Gain=C
  INT1 : UnitDelay  SampleTime=Ts
  INT2 : UnitDelay  SampleTime=Ts
  INT3 : UnitDelay  SampleTime=Ts
  Saturation{,1..4} (5 alike) : Saturate  UpperLimit=SAT  LowerLimit=-SAT
  OUT1 : Outport
  OUT2 : Outport  Port=2
  OUT3 : Outport  Port=3
  wires:
  SUB3/1 -> Add2/3
  INT1/1 -> Add2/1, OUT3/1
  INT2/1 -> OUT1/1, Add4/1, Add1/2
  Add4/1 -> Saturation/1
  SUB1/1 -> Add4/3, Add1/3
  IN/1 -> Gain/1, Gain2/1, Gain1/1
  Add1/1 -> Saturation1/1
  Gain/1 -> Add1/1
  Add2/1 -> Saturation2/1
  Saturation/1 -> INT2/1
  Saturation2/1 -> INT1/1
  INT3/1 -> OUT2/1, Add5/1, Add3/2
  Add5/1 -> Saturation3/1
  SUB2/1 -> Add5/3, Add3/3
  Add3/1 -> Saturation4/1
  Gain2/1 -> Add3/1
  Saturation3/1 -> INT3/1
  Saturation4/1 -> Add2/2
  Saturation1/1 -> Add5/2
  Gain1/1 -> Add4/2

== system AVIC_model/2値3次 NSDEM/NSDEM_3rd/INTEG4_4 ==
  IN : Inport
  SUB1 : Inport  Port=2
  SUB2 : Inport  Port=3
  SUB3 : Inport  Port=4
  Add{1..5} (5 alike) : Sum  Inputs=++-
  Gain : Gain  Gain=B2
  Gain1 : Gain  Gain=A
  Gain2 : Gain  Gain=C
  INT1 : UnitDelay  SampleTime=Ts
  INT2 : UnitDelay  SampleTime=Ts
  INT3 : UnitDelay  SampleTime=Ts
  Saturation{,1..4} (5 alike) : Saturate  UpperLimit=SAT  LowerLimit=-SAT
  OUT1 : Outport
  OUT2 : Outport  Port=2
  OUT3 : Outport  Port=3
  wires:
  SUB3/1 -> Add2/3
  INT1/1 -> Add2/1, OUT3/1
  INT2/1 -> OUT1/1, Add4/1, Add1/2
  Add4/1 -> Saturation/1
  SUB1/1 -> Add4/3, Add1/3
  IN/1 -> Gain/1, Gain2/1, Gain1/1
  Add1/1 -> Saturation1/1
  Gain/1 -> Add1/1
  Add2/1 -> Saturation2/1
  Saturation/1 -> INT2/1
  Saturation2/1 -> INT1/1
  INT3/1 -> OUT2/1, Add5/1, Add3/2
  Add5/1 -> Saturation3/1
  SUB2/1 -> Add5/3, Add3/3
  Add3/1 -> Saturation4/1
  Gain2/1 -> Add3/1
  Saturation3/1 -> INT3/1
  Saturation4/1 -> Add2/2
  Saturation1/1 -> Add5/2
  Gain1/1 -> Add4/2

== system AVIC_model/2値3次 NSDEM/NSDEM_3rd/INTEG4_5 ==
  IN : Inport
  SUB1 : Inport  Port=2
  SUB2 : Inport  Port=3
  SUB3 : Inport  Port=4
  Add{1..5} (5 alike) : Sum  Inputs=++-
  Gain : Gain  Gain=B2
  Gain1 : Gain  Gain=A
  Gain2 : Gain  Gain=C
  INT1 : UnitDelay  SampleTime=Ts
  INT2 : UnitDelay  SampleTime=Ts
  INT3 : UnitDelay  SampleTime=Ts
  Saturation{,1..4} (5 alike) : Saturate  UpperLimit=SAT  LowerLimit=-SAT
  OUT1 : Outport
  OUT2 : Outport  Port=2
  OUT3 : Outport  Port=3
  wires:
  SUB3/1 -> Add2/3
  INT1/1 -> Add2/1, OUT3/1
  INT2/1 -> OUT1/1, Add4/1, Add1/2
  Add4/1 -> Saturation/1
  SUB1/1 -> Add4/3, Add1/3
  IN/1 -> Gain/1, Gain2/1, Gain1/1
  Add1/1 -> Saturation1/1
  Gain/1 -> Add1/1
  Add2/1 -> Saturation2/1
  Saturation/1 -> INT2/1
  Saturation2/1 -> INT1/1
  INT3/1 -> OUT2/1, Add5/1, Add3/2
  Add5/1 -> Saturation3/1
  SUB2/1 -> Add5/3, Add3/3
  Add3/1 -> Saturation4/1
  Gain2/1 -> Add3/1
  Saturation3/1 -> INT3/1
  Saturation4/1 -> Add2/2
  Saturation1/1 -> Add5/2
  Gain1/1 -> Add4/2

== system AVIC_model/2値3次 NSDEM/NSDEM_3rd/INTEG4_6 ==
  IN : Inport
  SUB1 : Inport  Port=2
  SUB2 : Inport  Port=3
  SUB3 : Inport  Port=4
  Add{1..5} (5 alike) : Sum  Inputs=++-
  Gain : Gain  Gain=B2
  Gain1 : Gain  Gain=A
  Gain2 : Gain  Gain=C
  INT1 : UnitDelay  SampleTime=Ts
  INT2 : UnitDelay  SampleTime=Ts
  INT3 : UnitDelay  SampleTime=Ts
  Saturation{,1..4} (5 alike) : Saturate  UpperLimit=SAT  LowerLimit=-SAT
  OUT1 : Outport
  OUT2 : Outport  Port=2
  OUT3 : Outport  Port=3
  wires:
  SUB3/1 -> Add2/3
  INT1/1 -> Add2/1, OUT3/1
  INT2/1 -> OUT1/1, Add4/1, Add1/2
  Add4/1 -> Saturation/1
  SUB1/1 -> Add4/3, Add1/3
  IN/1 -> Gain/1, Gain2/1, Gain1/1
  Add1/1 -> Saturation1/1
  Gain/1 -> Add1/1
  Add2/1 -> Saturation2/1
  Saturation/1 -> INT2/1
  Saturation2/1 -> INT1/1
  INT3/1 -> OUT2/1, Add5/1, Add3/2
  Add5/1 -> Saturation3/1
  SUB2/1 -> Add5/3, Add3/3
  Add3/1 -> Saturation4/1
  Gain2/1 -> Add3/1
  Saturation3/1 -> INT3/1
  Saturation4/1 -> Add2/2
  Saturation1/1 -> Add5/2
  Gain1/1 -> Add4/2

== system AVIC_model/2値3次 NSDEM/NSDEM_3rd/INTEG4_7 ==
  IN : Inport
  SUB1 : Inport  Port=2
  SUB2 : Inport  Port=3
  SUB3 : Inport  Port=4
  Add{1..5} (5 alike) : Sum  Inputs=++-
  Gain : Gain  Gain=B2
  Gain1 : Gain  Gain=A
  Gain2 : Gain  Gain=C
  INT1 : UnitDelay  SampleTime=Ts
  INT2 : UnitDelay  SampleTime=Ts
  INT3 : UnitDelay  SampleTime=Ts
  Saturation{,1..4} (5 alike) : Saturate  UpperLimit=SAT  LowerLimit=-SAT
  OUT1 : Outport
  OUT2 : Outport  Port=2
  OUT3 : Outport  Port=3
  wires:
  SUB3/1 -> Add2/3
  INT1/1 -> Add2/1, OUT3/1
  INT2/1 -> OUT1/1, Add4/1, Add1/2
  Add4/1 -> Saturation/1
  SUB1/1 -> Add4/3, Add1/3
  IN/1 -> Gain/1, Gain2/1, Gain1/1
  Add1/1 -> Saturation1/1
  Gain/1 -> Add1/1
  Add2/1 -> Saturation2/1
  Saturation/1 -> INT2/1
  Saturation2/1 -> INT1/1
  INT3/1 -> OUT2/1, Add5/1, Add3/2
  Add5/1 -> Saturation3/1
  SUB2/1 -> Add5/3, Add3/3
  Add3/1 -> Saturation4/1
  Gain2/1 -> Add3/1
  Saturation3/1 -> INT3/1
  Saturation4/1 -> Add2/2
  Saturation1/1 -> Add5/2
  Gain1/1 -> Add4/2

== system AVIC_model/2値3次 NSDEM/NSDEM_3rd/INTEG4_8 ==
  IN : Inport
  SUB1 : Inport  Port=2
  SUB2 : Inport  Port=3
  SUB3 : Inport  Port=4
  Add{1..5} (5 alike) : Sum  Inputs=++-
  Gain : Gain  Gain=B2
  Gain1 : Gain  Gain=A
  Gain2 : Gain  Gain=C
  INT1 : UnitDelay  SampleTime=Ts
  INT2 : UnitDelay  SampleTime=Ts
  INT3 : UnitDelay  SampleTime=Ts
  Saturation{,1..4} (5 alike) : Saturate  UpperLimit=SAT  LowerLimit=-SAT
  OUT1 : Outport
  OUT2 : Outport  Port=2
  OUT3 : Outport  Port=3
  wires:
  SUB3/1 -> Add2/3
  INT1/1 -> Add2/1, OUT3/1
  INT2/1 -> OUT1/1, Add4/1, Add1/2
  Add4/1 -> Saturation/1
  SUB1/1 -> Add4/3, Add1/3
  IN/1 -> Gain/1, Gain2/1, Gain1/1
  Add1/1 -> Saturation1/1
  Gain/1 -> Add1/1
  Add2/1 -> Saturation2/1
  Saturation/1 -> INT2/1
  Saturation2/1 -> INT1/1
  INT3/1 -> OUT2/1, Add5/1, Add3/2
  Add5/1 -> Saturation3/1
  SUB2/1 -> Add5/3, Add3/3
  Add3/1 -> Saturation4/1
  Gain2/1 -> Add3/1
  Saturation3/1 -> INT3/1
  Saturation4/1 -> Add2/2
  Saturation1/1 -> Add5/2
  Gain1/1 -> Add4/2

== system AVIC_model/2値3次 NSDEM/NSDEM_3rd/INTEG4_9 ==
  IN : Inport
  SUB1 : Inport  Port=2
  SUB2 : Inport  Port=3
  SUB3 : Inport  Port=4
  Add{1..5} (5 alike) : Sum  Inputs=++-
  Gain : Gain  Gain=B2
  Gain1 : Gain  Gain=A
  Gain2 : Gain  Gain=C
  INT1 : UnitDelay  SampleTime=Ts
  INT2 : UnitDelay  SampleTime=Ts
  INT3 : UnitDelay  SampleTime=Ts
  Saturation{,1..4} (5 alike) : Saturate  UpperLimit=SAT  LowerLimit=-SAT
  OUT1 : Outport
  OUT2 : Outport  Port=2
  OUT3 : Outport  Port=3
  wires:
  SUB3/1 -> Add2/3
  INT1/1 -> Add2/1, OUT3/1
  INT2/1 -> OUT1/1, Add4/1, Add1/2
  Add4/1 -> Saturation/1
  SUB1/1 -> Add4/3, Add1/3
  IN/1 -> Gain/1, Gain2/1, Gain1/1
  Add1/1 -> Saturation1/1
  Gain/1 -> Add1/1
  Add2/1 -> Saturation2/1
  Saturation/1 -> INT2/1
  Saturation2/1 -> INT1/1
  INT3/1 -> OUT2/1, Add5/1, Add3/2
  Add5/1 -> Saturation3/1
  SUB2/1 -> Add5/3, Add3/3
  Add3/1 -> Saturation4/1
  Gain2/1 -> Add3/1
  Saturation3/1 -> INT3/1
  Saturation4/1 -> Add2/2
  Saturation1/1 -> Add5/2
  Gain1/1 -> Add4/2

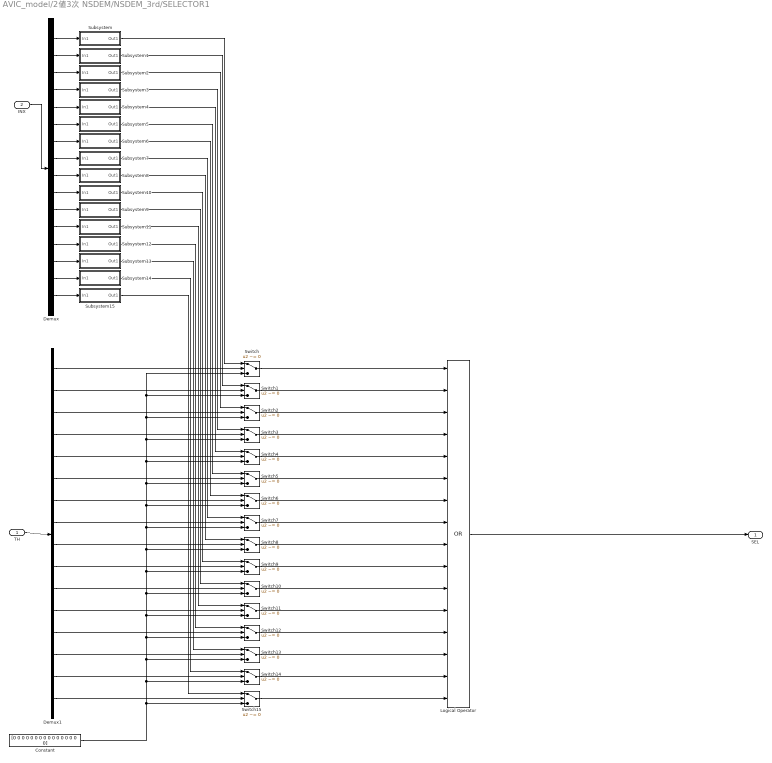
== system AVIC_model/2値3次 NSDEM/NSDEM_3rd/SELECTOR1 ==
  TH : Inport
  INX : Inport  Port=2
  Constant : Constant  Value=[0 0 0 0 0 0 0 0 0 0 0 0 0 0 0 0]
  Demux : Demux  Outputs=16
  Demux1 : Demux  Outputs=16
  Logical Operator : Logic  Operator=OR  Inputs=16  AllPortsSameDT=off  OutDataTypeStr=boolean
  Subsystem : Subsystem
  Subsystem1 : Subsystem
  Subsystem10 : Subsystem
  Subsystem11 : Subsystem
  Subsystem12 : Subsystem
  Subsystem13 : Subsystem
  Subsystem14 : Subsystem
  Subsystem15 : Subsystem
  Subsystem2 : Subsystem
  Subsystem3 : Subsystem
  Subsystem4 : Subsystem
  Subsystem5 : Subsystem
  Subsystem6 : Subsystem
  Subsystem7 : Subsystem
  Subsystem8 : Subsystem
  Subsystem9 : Subsystem
  Switch{,1..15} (16 alike) : Switch  Criteria=u2 ~= 0
  SEL : Outport
  wires:
  Logical Operator/1 -> SEL/1
  Demux1/8 -> Switch7/2
  Demux1/7 -> Switch6/2
  Demux1/6 -> Switch5/2
  Demux1/5 -> Switch4/2
  Demux1/4 -> Switch3/2
  Demux1/3 -> Switch2/2
  Demux1/2 -> Switch1/2
  Subsystem/1(Out1) -> Switch/1
  Demux1/1 -> Switch/2
  Demux/1 -> Subsystem/1(In1)
  INX/1 -> Demux/1
  TH/1 -> Demux1/1
  Demux1/9 -> Switch8/2
  Demux1/10 -> Switch9/2
  Demux1/11 -> Switch10/2
  Demux1/12 -> Switch11/2
  Demux1/13 -> Switch12/2
  Demux1/14 -> Switch13/2
  Demux1/15 -> Switch14/2
  Demux1/16 -> Switch15/2
  Subsystem1/1(Out1) -> Switch1/1
  Subsystem2/1(Out1) -> Switch2/1
  Subsystem3/1(Out1) -> Switch3/1
  Subsystem4/1(Out1) -> Switch4/1
  Subsystem5/1(Out1) -> Switch5/1
  Subsystem6/1(Out1) -> Switch6/1
  Subsystem7/1(Out1) -> Switch7/1
  Subsystem8/1(Out1) -> Switch8/1
  Subsystem10/1(Out1) -> Switch9/1
  Subsystem9/1(Out1) -> Switch10/1
  Subsystem11/1(Out1) -> Switch11/1
  Subsystem12/1(Out1) -> Switch12/1
  Subsystem13/1(Out1) -> Switch13/1
  Subsystem14/1(Out1) -> Switch14/1
  Subsystem15/1(Out1) -> Switch15/1
  Demux/2 -> Subsystem1/1(In1)
  Demux/3 -> Subsystem2/1(In1)
  Demux/4 -> Subsystem3/1(In1)
  Demux/5 -> Subsystem4/1(In1)
  Demux/6 -> Subsystem5/1(In1)
  Demux/7 -> Subsystem6/1(In1)
  Demux/8 -> Subsystem7/1(In1)
  Demux/9 -> Subsystem8/1(In1)
  Demux/10 -> Subsystem10/1(In1)
  Demux/11 -> Subsystem9/1(In1)
  Demux/12 -> Subsystem11/1(In1)
  Demux/13 -> Subsystem12/1(In1)
  Demux/14 -> Subsystem13/1(In1)
  Demux/15 -> Subsystem14/1(In1)
  Demux/16 -> Subsystem15/1(In1)
  Switch/1 -> Logical Operator/1
  Switch1/1 -> Logical Operator/2
  Switch2/1 -> Logical Operator/3
  Switch3/1 -> Logical Operator/4
  Switch4/1 -> Logical Operator/5
  Switch5/1 -> Logical Operator/6
  Switch6/1 -> Logical Operator/7
  Switch7/1 -> Logical Operator/8
  Switch8/1 -> Logical Operator/9
  Switch9/1 -> Logical Operator/10
  Switch10/1 -> Logical Operator/11
  Switch11/1 -> Logical Operator/12
  Switch12/1 -> Logical Operator/13
  Switch13/1 -> Logical Operator/14
  Switch14/1 -> Logical Operator/15
  Switch15/1 -> Logical Operator/16
  Constant/1 -> Switch4/3, Switch/3, Switch1/3, Switch2/3, Switch3/3, Switch5/3, Switch6/3, Switch7/3, Switch8/3, Switch9/3, Switch10/3, Switch11/3, Switch12/3, Switch13/3, Switch14/3, Switch15/3
